simulink model "Blinker_steuerung_2"  (R2015b)
settings: Solver=FixedStepAuto  StartTime=0.0  StopTime=inf  FixedStep=0.001  RelTol=1e-3
settings Model: Creator=guch0001  LastModifiedBy=scco1019

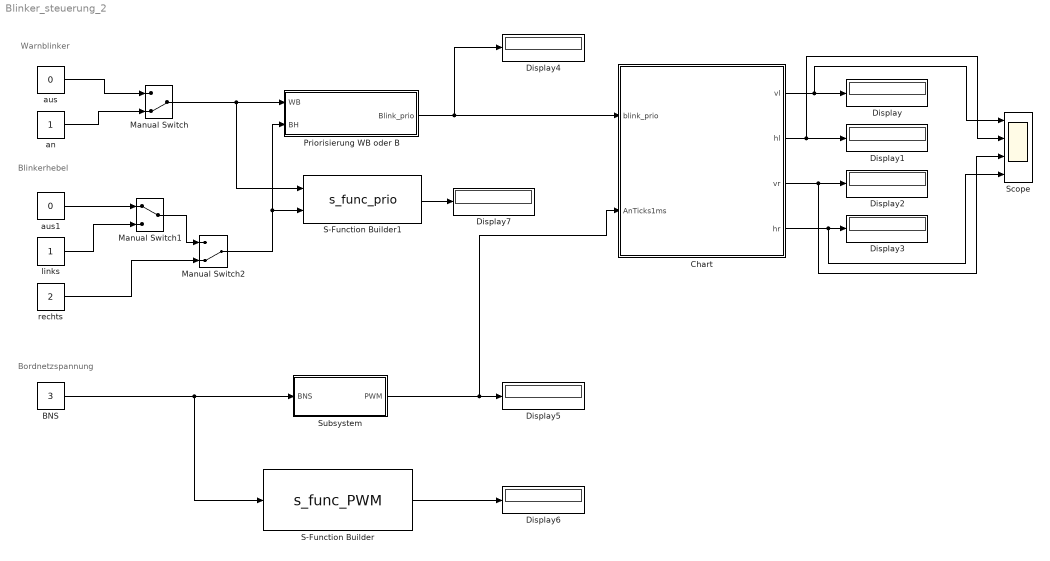
== system Blinker_steuerung_2 ==
  note: Bordnetzspannung
  note: Warnblinker
  note: Blinkerhebel
  BNS : Constant  Value=3
  Chart : Stateflow chart  TreatAsAtomicUnit=on
  Display{,1..7} (8 alike) : Display
  Manual Switch : ManualSwitch  CurrentSetting=0
  Manual Switch1 : ManualSwitch
  Manual Switch2 : ManualSwitch  CurrentSetting=0
  Priorisierung WB oder B : Subsystem
  S-Function Builder : S-Function  InitFcn=try, set_param(gcb,'FunctionName','s_func_PWM'), end  FunctionName=s_func_PWM  SFunctionModules=s_func_PWM_wrapper  SFunctionDeploymentMode=off  EnableBusSupport=off  mask(S-Function Builder){}
      mask help: Simulink:masks:SFunctionBuilder_MD
      mask init:
      | val = [[.9  0.75 0.75 1 1 .9 .9 1]',[1 1 0.75 0.75 .9 .9 1 .9]'];try , sys = get_param(gcb,'SfunBuilderFcnName');if isempty(sys), sys = get_param(gcb,'FunctionName'); end,catch, sys = get_param(gcb,'FunctionName'); end
      settings: CopyFcn=set_param(gcbh,'LinkStatus','none')  PreSaveFcn=try, set_param(gcb,'FunctionName','s_func_PWM'), end  OpenFcn=sfunctionwizard(gcbh)
      mask Display: plot(val(:,1),val(:,2)),disp(sys), port_label('input',1,'BNS'), port_label('output',1,'PWM')
  S-Function Builder1 : S-Function  InitFcn=try, set_param(gcb,'FunctionName','s_func_prio'), end  FunctionName=s_func_prio  SFunctionModules=s_func_prio_wrapper  SFunctionDeploymentMode=off  EnableBusSupport=off  mask(S-Function Builder){}
      mask help: Simulink:masks:SFunctionBuilder_MD
      mask init: same as Blinker_steuerung_2/S-Function Builder
      settings: CopyFcn=set_param(gcbh,'LinkStatus','none')  PreSaveFcn=try, set_param(gcb,'FunctionName','s_func_prio'), end  OpenFcn=sfunctionwizard(gcbh)
      mask Display: plot(val(:,1),val(:,2)),disp(sys), port_label('input',1,'WB'), port_label('input',2,'BH'), port_label('output',1,'Blink_prio')
  Scope : Scope  NumInputPorts=4
  Subsystem : Subsystem
  an : Constant
  aus : Constant  Value=0
  aus1 : Constant  Value=0
  links : Constant
  rechts : Constant  Value=2
  wires:
  aus/1 -> Manual Switch/1
  an/1 -> Manual Switch/2
  aus1/1 -> Manual Switch1/1
  links/1 -> Manual Switch1/2
  rechts/1 -> Manual Switch2/2
  Manual Switch1/1 -> Manual Switch2/1
  Manual Switch/1 -> S-Function Builder1/1, Priorisierung WB oder B/1(WB)
  Manual Switch2/1 -> S-Function Builder1/2, Priorisierung WB oder B/2(BH)
  Priorisierung WB oder B/1("Blink_prio ") -> Display4/1, Chart/1(blink_prio)
  Chart/4(hr) -> Scope/4, Display3/1
  Chart/1(vl) -> Scope/1, Display/1
  Chart/2(hl) -> Display1/1, Scope/2
  Chart/3(vr) -> Scope/3, Display2/1
  BNS/1 -> S-Function Builder/1, Subsystem/1(BNS)
  Subsystem/1(PWM) -> Chart/2(AnTicks1ms), Display5/1
  S-Function Builder/1 -> Display6/1
  S-Function Builder1/1 -> Display7/1

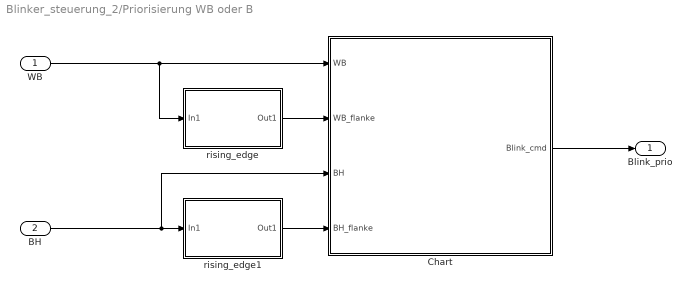
== system Blinker_steuerung_2/Priorisierung WB oder B ==
  WB : Inport
  BH : Inport  Port=2
  Chart : Stateflow chart  TreatAsAtomicUnit=on
  rising_edge : Subsystem
  rising_edge1 : Subsystem
  "Blink_prio " : Outport
  wires:
  BH/1 -> Chart/3(BH), rising_edge1/1(In1)
  WB/1 -> Chart/1(WB), rising_edge/1(In1)
  rising_edge/1(Out1) -> Chart/2(WB_flanke)
  rising_edge1/1(Out1) -> Chart/4(BH_flanke)
  Chart/1(Blink_cmd) -> "Blink_prio "/1

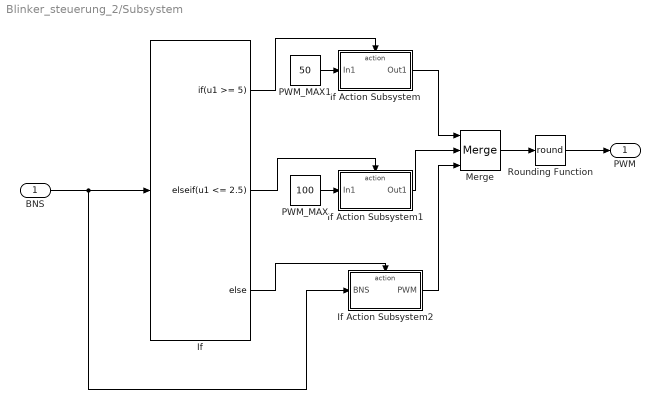
== system Blinker_steuerung_2/Subsystem ==
  BNS : Inport
  If : If  IfExpression=u1 >= 5  ElseIfExpressions=u1 <= 2.5
  If Action Subsystem : Subsystem  TreatAsAtomicUnit=on
  If Action Subsystem1 : Subsystem  TreatAsAtomicUnit=on
  If Action Subsystem2 : Subsystem  TreatAsAtomicUnit=on
  Merge : Merge  Inputs=3
  PWM_MAX : Constant  Value=100
  PWM_MAX1 : Constant  Value=50
  Rounding Function : Rounding  Operator=round
  PWM : Outport
  wires:
  BNS/1 -> If Action Subsystem2/1("BNS "), If/1
  If/1 -> If Action Subsystem/Action
  If Action Subsystem/1(Out1) -> Merge/1
  If/2 -> If Action Subsystem1/Action
  If Action Subsystem1/1(Out1) -> Merge/2
  If/3 -> If Action Subsystem2/Action
  If Action Subsystem2/1(PWM) -> Merge/3
  Merge/1 -> Rounding Function/1
  Rounding Function/1 -> PWM/1
  PWM_MAX/1 -> If Action Subsystem1/1(In1)
  PWM_MAX1/1 -> If Action Subsystem/1(In1)

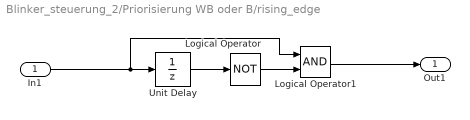
== system Blinker_steuerung_2/Priorisierung WB oder B/rising_edge ==
  In1 : Inport
  Logical Operator : Logic  Operator=NOT  AllPortsSameDT=off  OutDataTypeStr=boolean
  Logical Operator1 : Logic  AllPortsSameDT=off  OutDataTypeStr=boolean
  Unit Delay : UnitDelay  SampleTime=-1
  Out1 : Outport
  wires:
  In1/1 -> Logical Operator1/1, Unit Delay/1
  Unit Delay/1 -> Logical Operator/1
  Logical Operator/1 -> Logical Operator1/2
  Logical Operator1/1 -> Out1/1

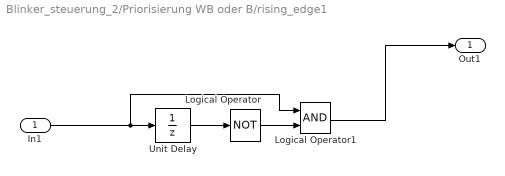
== system Blinker_steuerung_2/Priorisierung WB oder B/rising_edge1 ==
  In1 : Inport
  Logical Operator : Logic  Operator=NOT  AllPortsSameDT=off  OutDataTypeStr=boolean
  Logical Operator1 : Logic  AllPortsSameDT=off  OutDataTypeStr=boolean
  Unit Delay : UnitDelay  SampleTime=-1
  Out1 : Outport
  wires:
  Logical Operator1/1 -> Out1/1
  Logical Operator/1 -> Logical Operator1/2
  Unit Delay/1 -> Logical Operator/1
  In1/1 -> Unit Delay/1, Logical Operator1/1

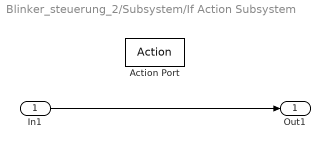
== system Blinker_steuerung_2/Subsystem/If Action Subsystem ==
  In1 : Inport
  Action Port : ActionPort  ActionType=then
  Out1 : Outport
  wires:
  In1/1 -> Out1/1

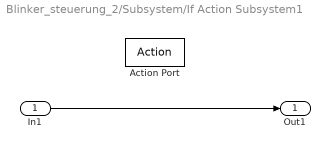
== system Blinker_steuerung_2/Subsystem/If Action Subsystem1 ==
  In1 : Inport
  Action Port : ActionPort  ActionType=elseif
  Out1 : Outport
  wires:
  In1/1 -> Out1/1

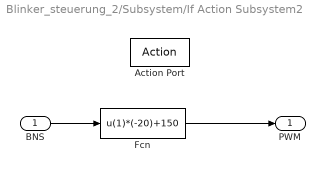
== system Blinker_steuerung_2/Subsystem/If Action Subsystem2 ==
  "BNS " : Inport
  Action Port : ActionPort  ActionType=else
  Fcn : Fcn  Expr=u(1)*(-20)+150
  PWM : Outport
  wires:
  "BNS "/1 -> Fcn/1
  Fcn/1 -> PWM/1

== stateflow chart Blinker_steuerung_2/Chart ==
  state AUS/
    entry:  vl=0; hl=0; vr=0; hr=0;
  state RECHTS/
    entry: counter1ms=mod(counter1ms+1,100);
  state LINKS/
    entry: counter1ms=mod(counter1ms+1,100);
  state WB/
    entry: counter1ms=mod(counter1ms+1,100);
  (default) -> AUS : {counter100ms=0;
      |  counter1ms=0;}
  AUS -> LINKS [order 3] : [blink_prio==1]{ANZEIT=AnTicks1ms;}
  AUS -> RECHTS [order 1] : [blink_prio==2]{ANZEIT=AnTicks1ms;}
  (junction 24) -> AUS [order 4]
  (junction 40) -> AUS [order 4]
  AUS -> WB [order 2] : [blink_prio==3]{ANZEIT=AnTicks1ms;}
  (junction 46) -> AUS [order 4]
  RECHTS -> RECHTS [order 3] : {vl=0;hl=0;vr=0;hr=0;}
  LINKS -> LINKS [order 3] : {vl=0;hl=0;vr=0;hr=0;}
  (junction 24) -> RECHTS [order 1] : [(blink_prio==2) && (counter100ms>9)]
      | {counter100ms=0;}
  (junction 24) -> LINKS [order 3] : [blink_prio==1]
      | {counter100ms=counter100ms+1;}
  RECHTS -> (junction 40) [order 1] : [counter1ms==0]
      | {ANZEIT=AnTicks1ms;}
  LINKS -> (junction 24) [order 1] : [counter1ms==0]
      | {ANZEIT=AnTicks1ms;}
  (junction 24) -> WB [order 2] : [(blink_prio==3) && (counter100ms>9)]
      | {counter100ms=0;}
  (junction 40) -> LINKS [order 3] : [(blink_prio==1) && (counter100ms>9)]
      | {counter100ms=0;}
  (junction 40) -> RECHTS [order 1] : [blink_prio==2]
      | {counter100ms=counter100ms+1;}
  (junction 40) -> WB [order 2] : [(blink_prio==3) && (counter100ms>9)]
      | {counter100ms=0;}
  (junction 46) -> RECHTS [order 2] : [(blink_prio==2) && (counter100ms>9)]
      | {counter100ms=0;}
  RECHTS -> RECHTS [order 2] : [(counter1ms<=ANZEIT)&&(mod(counter100ms,10)<5)]
      | {vl=0;hl=0;vr=1;hr=1;}
  (junction 46) -> LINKS [order 3] : [(blink_prio==1) && (counter100ms>9)]
      | {counter100ms=0;}
  LINKS -> LINKS [order 2] : [(counter1ms<=ANZEIT)&&(mod(counter100ms,10)<5)]
      | {vl=1;hl=1;vr=0;hr=0;}
  (junction 46) -> WB [order 1] : [blink_prio==3]
      | {counter100ms=counter100ms+1;}
  WB -> (junction 46) [order 1] : [counter1ms==0]
      | {ANZEIT=AnTicks1ms;}
  WB -> WB [order 3] : {vl=0;hl=0;vr=0;hr=0;}
  WB -> WB [order 2] : [(counter1ms<=ANZEIT)&&(mod(counter100ms,10)<5)]
      | {vl=1;hl=1;vr=1;hr=1;}
  data: blink_prio input; vl output; hl output; vr output; hr output; AnTicks1ms input; ANZEIT local; counter1ms local; counter100ms local

== stateflow chart Blinker_steuerung_2/Priorisierung WB oder B/Chart ==
  state RB_hat_Prio/
  state WB_hat_Prio/
  (default) -> RB_hat_Prio
  RB_hat_Prio -> (junction 16) [order 2]
  (junction 16) -> RB_hat_Prio [order 1] : [BH==1]{Blink_cmd=1;}
  (junction 16) -> RB_hat_Prio [order 2] : [BH==2]{Blink_cmd=2;}
  (junction 16) -> RB_hat_Prio [order 4] : {Blink_cmd=0;}
  (junction 16) -> RB_hat_Prio [order 3] : [WB==1]{Blink_cmd=3;}
  WB_hat_Prio -> RB_hat_Prio [order 1] : [BH_flanke==1]
  RB_hat_Prio -> WB_hat_Prio [order 1] : [WB_flanke==1]
  WB_hat_Prio -> (junction 4) [order 2]
  (junction 4) -> WB_hat_Prio [order 1] : [WB==1]{Blink_cmd=3;}
  (junction 4) -> WB_hat_Prio [order 4] : {Blink_cmd=0;}
  (junction 4) -> WB_hat_Prio [order 3] : [BH==2]{Blink_cmd=2;}
  (junction 4) -> WB_hat_Prio [order 2] : [BH==1]{Blink_cmd=1;}
  data: WB input; WB_flanke input; BH input; BH_flanke input; Blink_cmd output
